simulink model "pendulum"  (R2021a)
settings: Solver=VariableStepAuto  StartTime=0.0  StopTime=100  RelTol=1e-3
StartFcn:
  | AnimationInit;
values from neighbouring files (symbols this model uses):
  figId = gcf().Number    [AnimationInit.m]
libraries: aerolibanimutils x1, vrlib x1
settings Model: Creator=l.ribeiro-lustosa  LastModifiedBy=l.ribeiro-lustosa

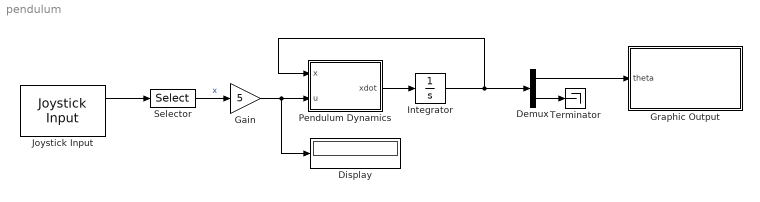
== system pendulum ==
  Demux : Demux  Outputs=2
  Display : Display
  Gain : Gain  Gain=5
  Graphic Output : Subsystem
  Integrator : Integrator  InitialCondition=[175*pi/180;0]
  Joystick Input : vrlib/Joystick Input  joyid=1  adjustports=on  forcefeed=off
  Pendulum Dynamics : MATLAB Function  TreatAsAtomicUnit=on
  Selector : Selector  IndexOptions=Index vector (dialog)  Indices=3  OutputSizes=1
  Terminator : Terminator
  wires:
  Pendulum Dynamics/1(xdot) -> Integrator/1
  Integrator/1 -> Demux/1, Pendulum Dynamics/1(x)
  Demux/2 -> Terminator/1
  Joystick Input/1 -> Selector/1
  Selector/1 -> Gain/1  "x"
  Gain/1 -> Display/1, Pendulum Dynamics/2(u)
  Demux/1 -> Graphic Output/1(theta)

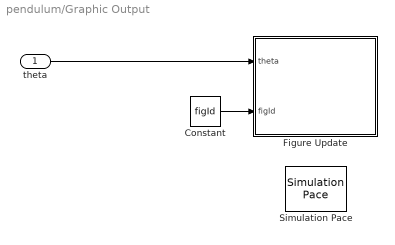
== system pendulum/Graphic Output ==
  theta : Inport
  Constant : Constant  Value=figId
  Figure Update : MATLAB Function  TreatAsAtomicUnit=on
  Simulation Pace : aerolibanimutils/Simulation Pace  SimulationPace=1  SleepMode=Auto  OutputPaceError=off  SampleTime=1/30
  wires:
  Constant/1 -> Figure Update/2(figId)
  theta/1 -> Figure Update/1(theta)

== matlab function pendulum/Pendulum Dynamics ==
  data: x input; xdot output; u input
function xdot = pendulum(x,u)

L = 1;
g = 10;
b = 0.5;

xdot = zeros(2,1);
xdot(1) = x(2);
xdot(2) = -g/L*sin(x(1)) - b*x(2) + u;

== matlab function pendulum/Graphic Output/Figure Update ==
  data: theta input; figId input
function updateFigure(theta, figId)

L = 1;

% drawing rod
dx = [0;L*sin(theta)];
dy = [0;-L*cos(theta)];
UpdatePlot(figId,'rod',dx,dy);
% drawing pendulum ball
dx = [L*sin(theta)];
dy = [-L*cos(theta)];
UpdatePlot(figId,'ball',dx,dy);

drawnow;

end

function UpdatePlot(hFig, plotTag, xData, yData)
    plotTarget = findobj(hFig, 'Tag', plotTag);
    set(plotTarget, 'XData', xData);
    set(plotTarget, 'YData', yData);
end
